simulink model "squad"  (R2012b)
settings: Solver=ode3  StartTime=0.0  StopTime=10.0  FixedStep=dt  RelTol=1e-3
values from neighbouring files (symbols this model uses):
  ampl = 5    [param.m]
  dt = 0.00005    (= 5e-05)    [param.m]
  freq = 5000    [param.m]
  T = 0.15    [param.m]
undefined symbols (not defined in the file or in its folder): DiscIntNeverNeededParam, random
libraries: commchan3 x1
settings Model: Creator=mishuk  LastModifiedBy=mishuk

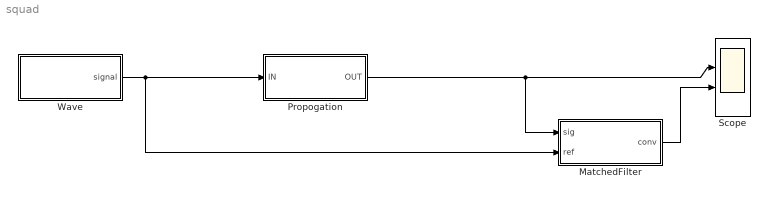
== system squad ==
  MatchedFilter : Subsystem
  Propogation : Subsystem
  Scope : Scope  NumInputPorts=4
      settings: TimeRange=1  YMin=-1~-4~-0.008~-5  YMax=1~6~0.006~5
  Wave : Subsystem
  wires:
  Propogation/1(OUT) -> Scope/2, MatchedFilter/1(sig)
  MatchedFilter/1(conv) -> Scope/3
  Wave/1(signal) -> Propogation/1(IN), MatchedFilter/2(ref)

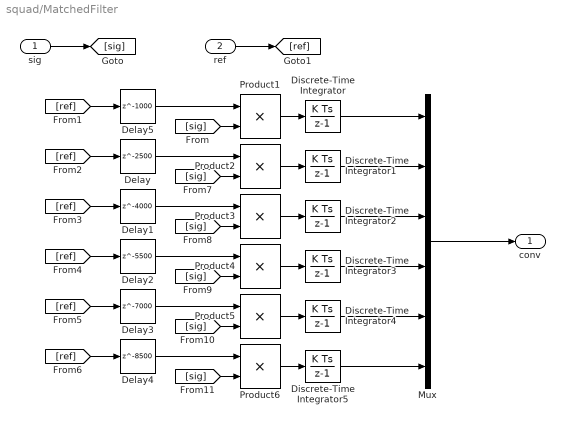
== system squad/MatchedFilter ==
  sig : Inport
  ref : Inport  Port=2
  Delay : Delay  DelayLength=2500
  Delay1 : Delay  DelayLength=4000
  Delay2 : Delay  DelayLength=5500
  Delay3 : Delay  DelayLength=7000
  Delay4 : Delay  DelayLength=8500
  Delay5 : Delay  DelayLength=1000
  Discrete-Time Integrator{,1..5} (6 alike) : DiscreteIntegrator  SampleTime=dt  ICPrevOutput=DiscIntNeverNeededParam  ICPrevScaledInput=DiscIntNeverNeededParam
  Mux : Mux  Inputs=6
  Product{1..6} (6 alike) : Product  RndMeth=Zero
  conv : Outport
  wires:
  Product1/1 -> Discrete-Time Integrator/1
  Mux/1 -> conv/1
  sig/1 -> [sig]
  ref/1 -> [ref]
  Delay5/1 -> Product1/1
  [sig] -> Product1/2
  [ref] -> Delay5/1
  [ref] -> Delay/1
  [ref] -> Delay1/1
  [ref] -> Delay2/1
  [ref] -> Delay3/1
  [ref] -> Delay4/1
  Product2/1 -> Discrete-Time Integrator1/1
  Delay/1 -> Product2/1
  [sig] -> Product2/2
  Product3/1 -> Discrete-Time Integrator2/1
  [sig] -> Product3/2
  Product4/1 -> Discrete-Time Integrator3/1
  [sig] -> Product4/2
  Product5/1 -> Discrete-Time Integrator4/1
  [sig] -> Product5/2
  Product6/1 -> Discrete-Time Integrator5/1
  [sig] -> Product6/2
  Delay1/1 -> Product3/1
  Delay2/1 -> Product4/1
  Delay3/1 -> Product5/1
  Delay4/1 -> Product6/1
  Discrete-Time Integrator/1 -> Mux/1
  Discrete-Time Integrator1/1 -> Mux/2
  Discrete-Time Integrator2/1 -> Mux/3
  Discrete-Time Integrator3/1 -> Mux/4
  Discrete-Time Integrator4/1 -> Mux/5
  Discrete-Time Integrator5/1 -> Mux/6

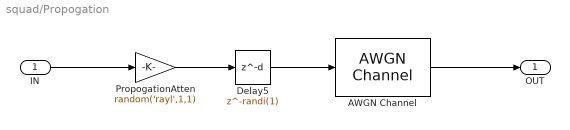
== system squad/Propogation ==
  IN : Inport
  AWGN Channel : commchan3/AWGN Channel  InputProcessing=Columns as channels (frame based)  seed=67  noiseMode=Variance from mask  EbNodB=10  EsNodB=10  SNRdB=0  bitsPerSym=1  Ps=0.01  Tsym=1  variance=noiseVariance
  Delay5 : Delay  DelayLength=randi(1)
  PropogationAtten : Gain  Gain=random('rayl',1,1)
  OUT : Outport
  wires:
  PropogationAtten/1 -> Delay5/1
  Delay5/1 -> AWGN Channel/1
  IN/1 -> PropogationAtten/1
  AWGN Channel/1 -> OUT/1

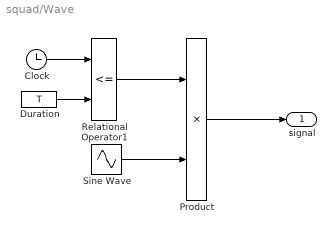
== system squad/Wave ==
  Clock : Clock
  Duration : Constant  Value=T
  Product : Product  RndMeth=Zero
  Relational Operator1 : RelationalOperator  Operator=<=  OutDataTypeStr=boolean
  Sine Wave : Sin  Amplitude=ampl  Frequency=2*pi*freq  Phase=2*pi*rand(1)  SampleTime=dt
  signal : Outport
  wires:
  Duration/1 -> Relational Operator1/2
  Product/1 -> signal/1
  Clock/1 -> Relational Operator1/1
  Sine Wave/1 -> Product/2
  Relational Operator1/1 -> Product/1
